simulink model "realfunction"  (R2019a)
settings: Solver=VariableStepAuto  StartTime=0.0  StopTime=10.0  RelTol=1e-3
settings Model: Creator=zq001  LastModifiedBy=zq001

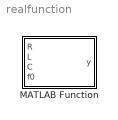
== system realfunction ==
  MATLAB Function : MATLAB Function  TreatAsAtomicUnit=on

== matlab function realfunction/MATLAB Function ==
  data: R input; L input; C input; y output; f0 input
function y = fcn(R,L,C,f0)

% CIRCUIT:
% |--R---L-----|       1/(L+R)    1./(1j*w0*x(2)*u2+x(1))
% |              |
% |------Cparasitic------|         Cp    1j*w0*x(3)*u1
% |              |
% |-------Cspacing----|             Cs   1j*w0*x(4)*u1
%
% parameter meaning:
% a(1)--->R
% a(2)--->L
% a(3)--->Cp
% a(4)--->Cs
% 
% F = Zeq = 1/((1/R+jwL) + jwCp + jwCs)
w0 = 2*pi*f0;
u1 = 1;
u2 = 1;
Zcal = real(1./( (1./(1j*w0*L*u2+R)) + 1j*w0*C*u1 ));
end
